simulink model "control_graph"  (R2018a)
settings: Solver=VariableStepAuto  StartTime=0.0  StopTime=10.0  RelTol=1e-3
settings Model: Creator=28718  LastModifiedBy=28718

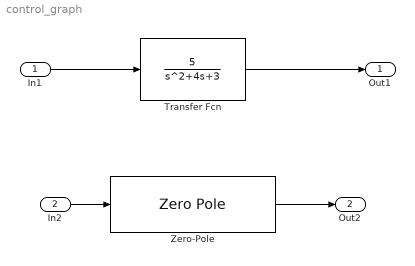
== system control_graph ==
  In1 : Inport
  In2 : Inport  Port=2
  Transfer Fcn : TransferFcn  Numerator=[5]  Denominator=[1 4 3]
  Zero-Pole : ZeroPole  Zeros=[-2]  Poles=[-1 -2 -3]  Gain=[5]
  Out1 : Outport
  Out2 : Outport  Port=2
  wires:
  In1/1 -> Transfer Fcn/1
  Transfer Fcn/1 -> Out1/1
  In2/1 -> Zero-Pole/1
  Zero-Pole/1 -> Out2/1
